simulink subsystem "bmi_auto_calibration"  (R2023b)
settings: Solver=VariableStepAuto  StartTime=0.0  StopTime=10.0  RelTol=1e-3
values from neighbouring files (symbols this model uses):
  tvs =     [tvs_parameters.mat]
libraries: matrix_library x1, vrlib x1, dspstat3 x1
settings Model: Creator=Inver  LastModifiedBy=Inver

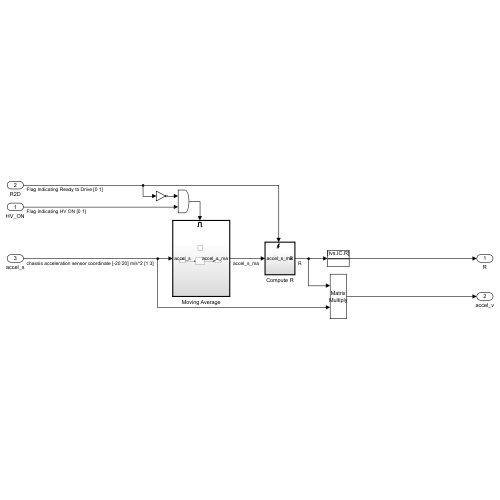
[thumbnail: Simulink's stored preview of the top-level diagram]
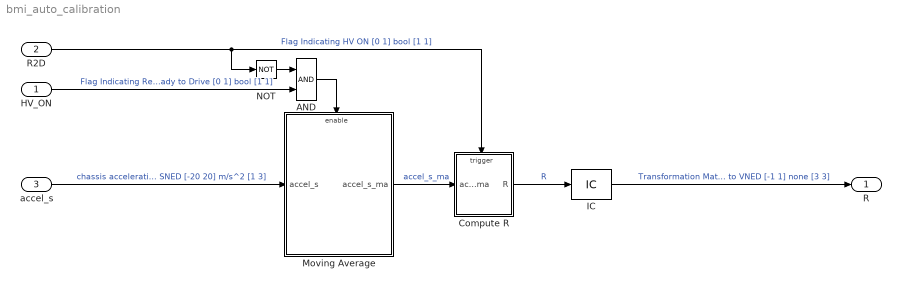
== system bmi_auto_calibration ==
  HV_ON : Inport
  R2D : Inport  Port=2
  accel_s : Inport  Port=3
  AND : Logic  IconShape=distinctive  AllPortsSameDT=off  OutDataTypeStr=boolean
  Compute R : Subsystem
  IC : InitialCondition  Value=tvs.IC.R
  Moving Average : Subsystem
  NOT : Logic  Operator=NOT  IconShape=distinctive  AllPortsSameDT=off  OutDataTypeStr=boolean
  R : Outport
  wires:
  NOT/1 -> AND/1
  R2D/1 -> NOT/1, Compute R/Trigger  "Flag Indicating HV ON [0 1] bool [1 1]"
  Compute R/1(R) -> IC/1  "R"
  accel_s/1 -> Moving Average/1(accel_s)  "chassis acceleration SNED [-20 20] m/s^2 [1 3]"
  Moving Average/1(accel_s_ma) -> Compute R/1(accel_s_ma)  "accel_s_ma"
  HV_ON/1 -> AND/2  "Flag Indicating Ready to Drive [0 1] bool [1 1]"
  IC/1 -> R/1  "Transformation Matrix SNED to VNED [-1 1] none [3 3]"
  AND/1 -> Moving Average/Enable

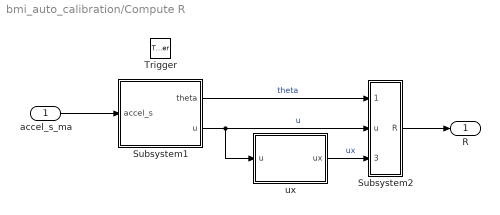
== system bmi_auto_calibration/Compute R ==
  accel_s_ma : Inport
  Trigger : TriggerPort  VariantControl=(inherit)  PortDimensions=1
  Subsystem1 : Subsystem
  Subsystem2 : Subsystem
  ux : MATLAB Function  TreatAsAtomicUnit=on
  R : Outport
  wires:
  ux/1(ux) -> Subsystem2/3(ux)  "ux"
  Subsystem1/2(u) -> ux/1(u), Subsystem2/2(u)  "u"
  Subsystem1/1(theta) -> Subsystem2/1(theta)  "theta"
  Subsystem2/1(R) -> R/1
  accel_s_ma/1 -> Subsystem1/1(accel_s)

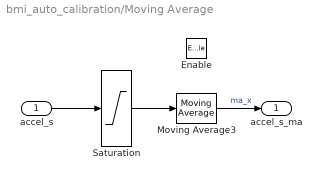
== system bmi_auto_calibration/Moving Average ==
  accel_s : Inport
  Enable : EnablePort
  Moving Average3 : dspstat3/Moving Average  Method=Sliding window  ForgettingFactorPort=off  SpecifyWindowLength=off  WindowLength=4  OverlapLength=3  AllowArbitraryInputLength=off  ForgettingFactor=0.9  SimulateUsing=Code generation
  Saturation : Saturate  UpperLimit=tvs.bounds.ub  LowerLimit=tvs.bounds.lb
  accel_s_ma : Outport
  wires:
  Saturation/1 -> Moving Average3/1
  Moving Average3/1 -> accel_s_ma/1  "ma_x"
  accel_s/1 -> Saturation/1

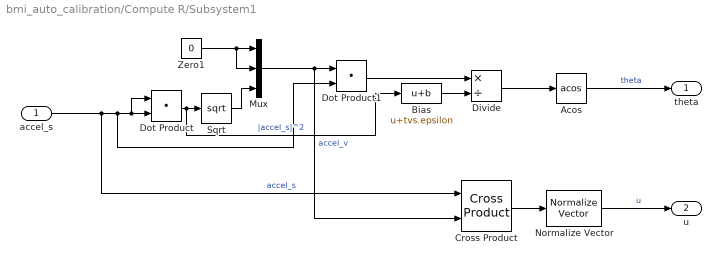
== system bmi_auto_calibration/Compute R/Subsystem1 ==
  accel_s : Inport  PortDimensions=[3 1]
  Acos : Trigonometry  Operator=acos
  Bias : Bias  Bias=tvs.epsilon  SaturateOnIntegerOverflow=off
  Cross Product : matrix_library/Cross Product
  Divide : Product  Inputs=*/
  Dot Product : DotProduct  OutDataTypeStr=Inherit: Inherit via internal rule
  Dot Product1 : DotProduct  OutDataTypeStr=Inherit: Inherit via internal rule
  Mux : Mux  Inputs=3
  Normalize Vector : vrlib/Utilities/Normalize Vector  maxzero=0
  Sqrt : Sqrt
  Zero1 : Constant  Value=0  OutDataTypeStr=Inherit: Inherit via back propagation
  theta : Outport
  u : Outport  Port=2
  wires:
  accel_s/1 -> Cross Product/1, Dot Product1/2, Dot Product/1, Dot Product/2  "accel_s"
  Cross Product/1 -> Normalize Vector/1
  Dot Product1/1 -> Divide/1
  Normalize Vector/1 -> u/1  "u"
  Dot Product/1 -> Bias/1, Sqrt/1  "|accel_s|^2"
  Sqrt/1 -> Mux/3
  Mux/1 -> Cross Product/2, Dot Product1/1  "accel_v"
  Zero1/1 -> Mux/2, Mux/1
  Divide/1 -> Acos/1
  Acos/1 -> theta/1  "theta"
  Bias/1 -> Divide/2

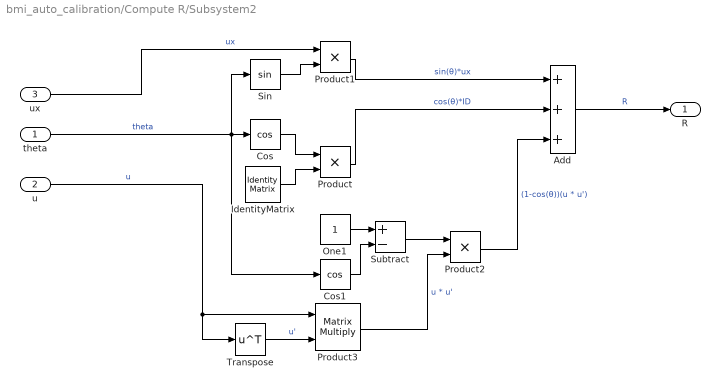
== system bmi_auto_calibration/Compute R/Subsystem2 ==
  theta : Inport
  u : Inport  Port=2
  ux : Inport  Port=3
  Add : Sum  Inputs=+++
  Cos : Trigonometry  Operator=cos
  Cos1 : Trigonometry  Operator=cos
  IdentityMatrix : IdentityMatrix  OutputDimensions=3  SampleTime=-1
  One1 : Constant  OutDataTypeStr=Inherit: Inherit via back propagation
  Product : Product
  Product1 : Product
  Product2 : Product
  Product3 : Product  Multiplication=Matrix(*)
  Sin : Trigonometry
  Subtract : Sum  Inputs=+-
  Transpose : Math  Operator=transpose
  R : Outport
  wires:
  theta/1 -> Cos1/1, Sin/1, Cos/1  "theta"
  Product/1 -> Add/2  "cos(θ)*ID"
  Cos1/1 -> Subtract/2
  Cos/1 -> Product/1
  Subtract/1 -> Product2/1
  ux/1 -> Product1/1  "ux"
  One1/1 -> Subtract/1
  IdentityMatrix/1 -> Product/2
  u/1 -> Product3/1, Transpose/1  "u"
  Sin/1 -> Product1/2
  Product1/1 -> Add/1  "sin(θ)*ux"
  Add/1 -> R/1  "R"
  Transpose/1 -> Product3/2  "u'"
  Product2/1 -> Add/3  "(1-cos(θ))(u * u')"
  Product3/1 -> Product2/2  "u * u'"

== matlab function bmi_auto_calibration/Compute R/ux ==
  data: u input size=[3 1]; ux output
function ux = fcn(u)

ux = [0 -u(3) u(2); u(3) 0 -u(1); -u(2) u(1) 0];
